simulink model "Tipo1VistaBloques"  (R2021b)
settings: Solver=VariableStepAuto  StartTime=0.0  StopTime=10.0  RelTol=1e-3
values from neighbouring files (symbols this model uses):
  A = sys.A    [RealEstadoObserServoTipo0.m]
  B = sys.B    [RealEstadoObserServoTipo0.m]
  C = sys.C    [RealEstadoObserServoTipo0.m]    (also in control 2 tf.mat = 0.0033)
  K = Khat(1:m-1)    [RealEstadoObserServoTipo0.m]
undefined symbols (not defined in the file or in its folder): ki
settings Model: Creator=Andre  LastModifiedBy=Andre

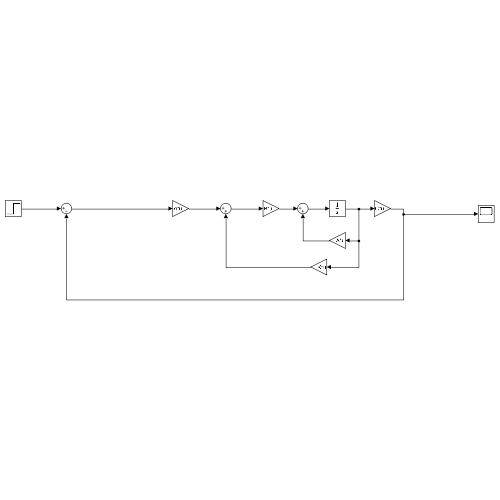
[thumbnail: Simulink's stored preview of the top-level diagram]
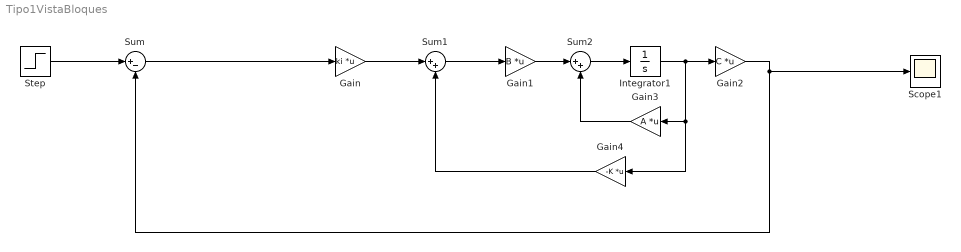
== system Tipo1VistaBloques ==
  Gain : Gain  Gain=ki  Multiplication=Matrix(K*u)
  Gain1 : Gain  Gain=B  Multiplication=Matrix(K*u)
  Gain2 : Gain  Gain=C  Multiplication=Matrix(K*u)
  Gain3 : Gain  Gain=A  Multiplication=Matrix(K*u)
  Gain4 : Gain  Gain=-K  Multiplication=Matrix(K*u)
  Integrator1 : Integrator
  Scope1 : Scope
  Step : Step  Time=0  SampleTime=0
  Sum : Sum  Inputs=|+-
  Sum1 : Sum  Inputs=|++
  Sum2 : Sum  Inputs=|++
  wires:
  Sum/1 -> Gain/1
  Step/1 -> Sum/1
  Integrator1/1 -> Gain4/1, Gain3/1, Gain2/1
  Gain2/1 -> Scope1/1, Sum/2
  Gain4/1 -> Sum1/2
  Gain3/1 -> Sum2/2
  Sum2/1 -> Integrator1/1
  Gain1/1 -> Sum2/1
  Sum1/1 -> Gain1/1
  Gain/1 -> Sum1/1
